simulink model "Difference_equation_model"  (R2020b)
settings: Solver=VariableStepAuto  StartTime=0.0  StopTime=10.0  RelTol=1e-3
settings Model: Creator=Training  LastModifiedBy=Training

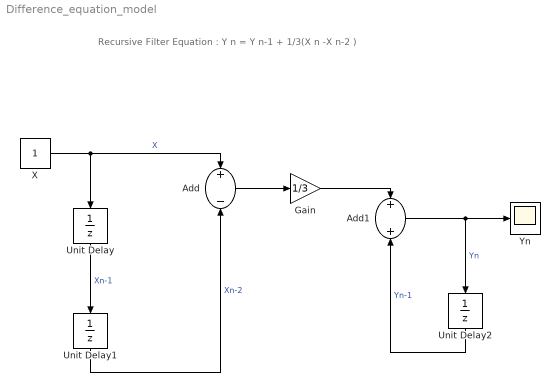
== system Difference_equation_model ==
  note: Recursive Filter Equation :
      |
      | Y n = Y n-1 + 1/3(X n -X n-2 )
  Add : Sum  Inputs=+-
  Add1 : Sum
  Gain : Gain  Gain=1/3
  Unit Delay : UnitDelay  SampleTime=-1  HasFrameUpgradeWarning=on
  Unit Delay1 : UnitDelay  SampleTime=-1  HasFrameUpgradeWarning=on
  Unit Delay2 : UnitDelay  SampleTime=-1  HasFrameUpgradeWarning=on
  X : Constant
  Yn : Scope
  wires:
  X/1 -> Unit Delay/1, Add/1  "X"
  Unit Delay/1 -> Unit Delay1/1  "Xn-1"
  Unit Delay1/1 -> Add/2  "Xn-2"
  Add/1 -> Gain/1
  Gain/1 -> Add1/1
  Add1/1 -> Unit Delay2/1, Yn/1  "Yn"
  Unit Delay2/1 -> Add1/2  "Yn-1"
